simulink model "example_SITL"  (R2018b)
settings: Solver=FixedStepAuto  StartTime=0.0  StopTime=inf  FixedStep=1/4000  RelTol=1e-3
values from neighbouring files (symbols this model uses):
  ddot_EulerAngles_steady = [0;0;0.1]    [ardupilot_sitl_example_init.m]    (also in init_exampleSITL.m)
  ddot_EulerAngles_unsteady = [0.1;0.05;0]    [ardupilot_sitl_example_init.m]    (also in init_exampleSITL.m)
  dot_V_Kb_unsteady = [4;0;0]    [ardupilot_sitl_example_init.m]    (also in init_exampleSITL.m)
  Phi_steady = 0.5    [ardupilot_sitl_example_init.m]    (also in init_exampleSITL.m)
  V_Kb_steady = 20    [ardupilot_sitl_example_init.m]    (also in init_exampleSITL.m)
libraries: axes_transformation_lib x2, simulink x2, ardupilot_sitl_lib x1, aerolibanimutils x1, sensors_lib x1
settings Model: SimulationMode=accelerator  Creator=yannic  LastModifiedBy=Yannic

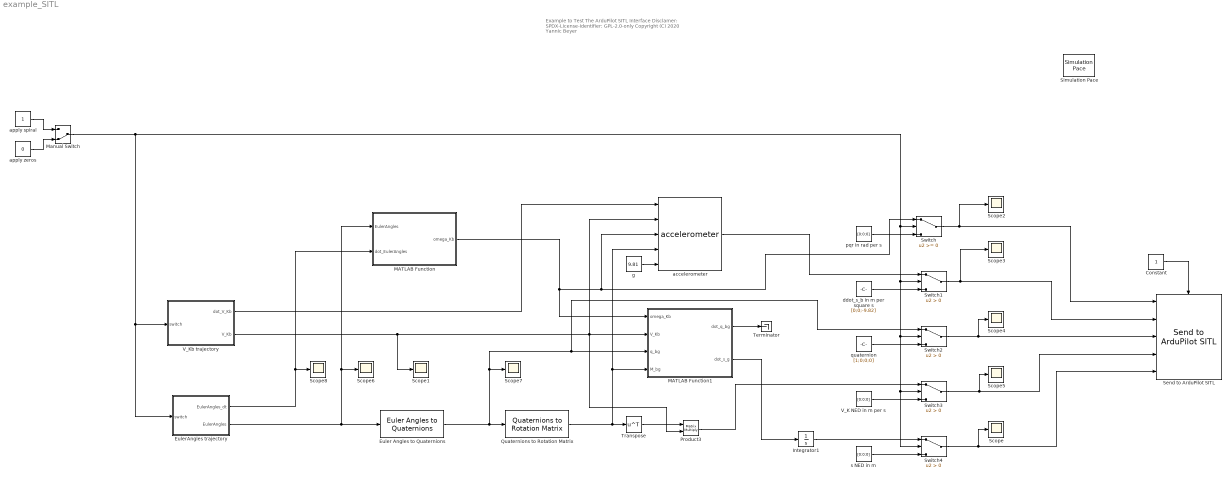
== system example_SITL ==
  note: Example to Test The ArduPilot SITL Interface
      |
      | Disclamer:
      | SPDX-License-Identifier: GPL-2.0-only
      |
      | Copyright (C) 2020 Yannic Beyer
  Constant : Constant
  Euler Angles to Quaternions : axes_transformation_lib/Euler Angles to Quaternions  SystemSampleTime=-1
      settings: SourceProductName=LADAC
  EulerAngles trajectory : Subsystem
  Integrator1 : Integrator
  MATLAB Function : MATLAB Function  TreatAsAtomicUnit=on
  MATLAB Function1 : MATLAB Function  TreatAsAtomicUnit=on
  Manual Switch : ManualSwitch  CurrentSetting=0
  Product3 : Product  Multiplication=Matrix(*)
  Quaternions to Rotation Matrix : axes_transformation_lib/Quaternions to Rotation Matrix  SystemSampleTime=-1
      settings: SourceProductName=LADAC
  Scope{,1..8} (9 alike) : Scope
  Send to ArduPilot SITL : ardupilot_sitl_lib/Send to ArduPilot SITL  IP='127.0.0.1'  Port=9003  sample_time=1/4000
      settings: SourceProductName=LADAC
  Simulation Pace : aerolibanimutils/Simulation Pace  SimulationPace=1  SleepMode=Auto  OutputPaceError=off  SampleTime=-1
  Switch : Switch
  Switch{1..4} (4 alike) : Switch  Criteria=u2 > Threshold
  Terminator : Terminator
  Transpose : Math  Operator=transpose  SaturateOnIntegerOverflow=on
  V_K NED in m per s : Constant  Value=[0;0;0]
  V_Kb trajectory : Subsystem
  accelerometer : sensors_lib/accelerometer  SystemSampleTime=-1
  apply spiral : Constant
  apply zeros : Constant  Value=0
  ddot_s_b in m per square s : Constant  Value=[0;0;-9.82]
  g : Constant  Value=9.81
  pqr in rad per s : Constant  Value=[0;0;0]
  quaternion : Constant  Value=[1;0;0;0]
  s NED in m : Constant  Value=[0;0;0]
  wires:
  Euler Angles to Quaternions/1 -> Scope7/1, Switch2/1, MATLAB Function1/3(q_bg), Quaternions to Rotation Matrix/1
  Switch3/1 -> Scope5/1, Send to ArduPilot SITL/4
  MATLAB Function1/2(dot_s_g) -> Integrator1/1
  MATLAB Function1/1(dot_q_bg) -> Terminator/1
  Switch4/1 -> Send to ArduPilot SITL/5, Scope/1
  Manual Switch/1 -> V_Kb trajectory/1(switch), EulerAngles trajectory/1(switch), Switch/2, Switch2/2, Switch3/2, Switch4/2, Switch1/2
  apply spiral/1 -> Manual Switch/1
  apply zeros/1 -> Manual Switch/2
  MATLAB Function/1(omega_Kb) -> MATLAB Function1/1(omega_Kb), Switch/1, accelerometer/3
  ddot_s_b in m per square s/1 -> Switch1/3
  accelerometer/1 -> Switch1/1
  quaternion/1 -> Switch2/3
  V_K NED in m per s/1 -> Switch3/3
  s NED in m/1 -> Switch4/3
  Transpose/1 -> Product3/1
  Product3/1 -> Switch3/1
  pqr in rad per s/1 -> Switch/3
  Quaternions to Rotation Matrix/1 -> accelerometer/4, MATLAB Function1/4(M_bg), Transpose/1
  Switch2/1 -> Send to ArduPilot SITL/3, Scope4/1
  Integrator1/1 -> Switch4/1
  Switch/1 -> Send to ArduPilot SITL/1, Scope2/1
  Switch1/1 -> Send to ArduPilot SITL/2, Scope3/1
  EulerAngles trajectory/2(EulerAngles) -> MATLAB Function/1(EulerAngles), Scope6/1, Euler Angles to Quaternions/1
  EulerAngles trajectory/1(EulerAngles_dt) -> MATLAB Function/2(dot_EulerAngles), Scope8/1
  V_Kb trajectory/2(V_Kb) -> Product3/2, MATLAB Function1/2(V_Kb), accelerometer/2, Scope1/1
  V_Kb trajectory/1(dot_V_Kb) -> accelerometer/1
  g/1 -> accelerometer/5
  Constant/1 -> Send to ArduPilot SITL/Enable

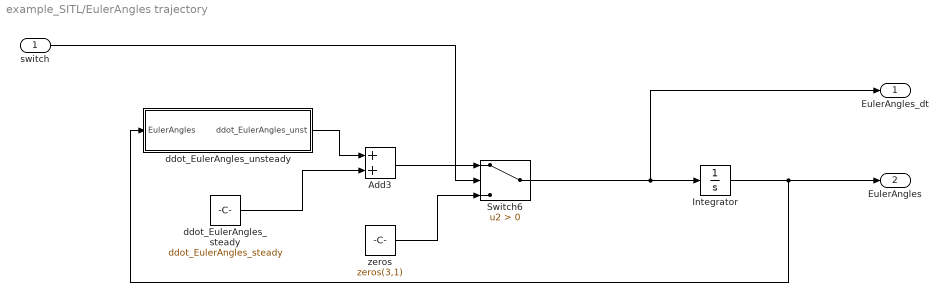
== system example_SITL/EulerAngles trajectory ==
  switch : Inport
  Add3 : Sum
  Integrator : Integrator  InitialCondition=[0;0;0]
  Switch6 : Switch  Criteria=u2 > Threshold
  ddot_EulerAngles_steady : Constant  Value=ddot_EulerAngles_steady
  ddot_EulerAngles_unsteady : Subsystem
  zeros : Constant  Value=zeros(3,1)
  EulerAngles_dt : Outport
  EulerAngles : Outport  Port=2
  wires:
  zeros/1 -> Switch6/3
  switch/1 -> Switch6/2
  ddot_EulerAngles_steady/1 -> Add3/2
  Switch6/1 -> EulerAngles_dt/1, Integrator/1
  Integrator/1 -> ddot_EulerAngles_unsteady/1(EulerAngles), EulerAngles/1
  Add3/1 -> Switch6/1
  ddot_EulerAngles_unsteady/1(ddot_EulerAngles_unst) -> Add3/1

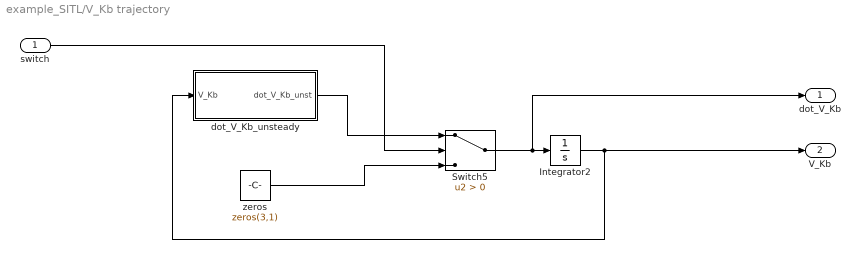
== system example_SITL/V_Kb trajectory ==
  switch : Inport
  Integrator2 : Integrator  InitialCondition=[0;0;0]
  Switch5 : Switch  Criteria=u2 > Threshold
  dot_V_Kb_unsteady : Subsystem
  zeros : Constant  Value=zeros(3,1)
  dot_V_Kb : Outport
  V_Kb : Outport  Port=2
  wires:
  switch/1 -> Switch5/2
  zeros/1 -> Switch5/3
  Switch5/1 -> dot_V_Kb/1, Integrator2/1
  Integrator2/1 -> dot_V_Kb_unsteady/1(V_Kb), V_Kb/1
  dot_V_Kb_unsteady/1(dot_V_Kb_unst) -> Switch5/1

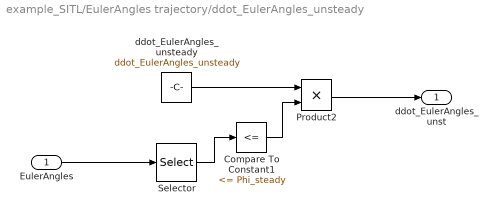
== system example_SITL/EulerAngles trajectory/ddot_EulerAngles_unsteady ==
  EulerAngles : Inport
  Compare To Constant1 : simulink/Logic and Bit Operations/Compare To Constant  relop=<=  const=Phi_steady  OutDataTypeStr=boolean
  Product2 : Product
  Selector : Selector  InputPortWidth=3  IndexOptions=Index vector (dialog)  Indices=1  OutputSizes=1
  ddot_EulerAngles_unsteady : Constant  Value=ddot_EulerAngles_unsteady
  ddot_EulerAngles_unst : Outport
  wires:
  EulerAngles/1 -> Selector/1
  Product2/1 -> ddot_EulerAngles_unst/1
  ddot_EulerAngles_unsteady/1 -> Product2/1
  Compare To Constant1/1 -> Product2/2
  Selector/1 -> Compare To Constant1/1

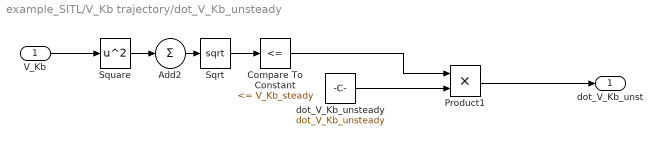
== system example_SITL/V_Kb trajectory/dot_V_Kb_unsteady ==
  V_Kb : Inport
  Add2 : Sum  Inputs=+
  Compare To Constant : simulink/Logic and Bit Operations/Compare To Constant  relop=<=  const=V_Kb_steady  OutDataTypeStr=boolean
  Product1 : Product
  Sqrt : Sqrt  SaturateOnIntegerOverflow=on
  Square : Math  Operator=square  SaturateOnIntegerOverflow=on
  dot_V_Kb_unsteady : Constant  Value=dot_V_Kb_unsteady
  dot_V_Kb_unst : Outport
  wires:
  V_Kb/1 -> Square/1
  Product1/1 -> dot_V_Kb_unst/1
  Compare To Constant/1 -> Product1/1
  dot_V_Kb_unsteady/1 -> Product1/2
  Add2/1 -> Sqrt/1
  Square/1 -> Add2/1
  Sqrt/1 -> Compare To Constant/1

== matlab function example_SITL/MATLAB Function1 ==
  data: omega_Kb input; dot_q_bg output; V_Kb input; q_bg input; M_bg input; dot_s_g output
function [ dot_q_bg, dot_s_g ] = ...
    fcn( omega_Kb, V_Kb, q_bg, M_bg )%#codegen
[ dot_q_bg, dot_s_g ] = ...
    rigidBodyKinematicsQuat( omega_Kb, V_Kb, q_bg, M_bg );
end

== matlab function example_SITL/MATLAB Function ==
  data: EulerAngles input; omega_Kb output; dot_EulerAngles input
function omega_Kb = fcn(EulerAngles,dot_EulerAngles)
%#codegen
    Theta = EulerAngles(1);
    Phi = EulerAngles(2);
    M = [ 1, 0, -sin(Theta); ...
        0, cos(Phi), sin(Phi)*cos(Theta); ...
        0, -sin(Phi), cos(Phi)*cos(Theta) ];
    omega_Kb = M * dot_EulerAngles;
end
